simulink subsystem "VDBS14DOF"  (R2022a)
settings: Solver=VariableStepAuto  StartTime=0.0  StopTime=10.0  RelTol=1e-3
undefined symbols (not defined in the file or in its folder): egoActorID, max_ac, max_dc
settings Model: Creator=The MathWorks, Inc.  LastModifiedBy=The MathWorks, Inc.
settings SolverCC: MaxZcPerStep=1
settings DebuggingCC: UnconnectedInputMsg=warning  UnconnectedOutputMsg=warning  UnconnectedLineMsg=warning
settings RTWCC: DLArmComputeVersion=19.05

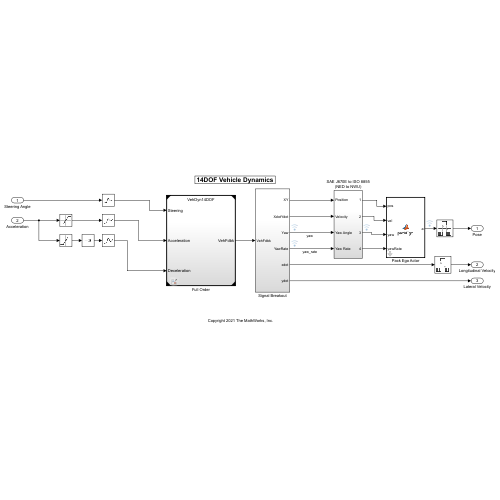
[thumbnail: Simulink's stored preview of the top-level diagram]
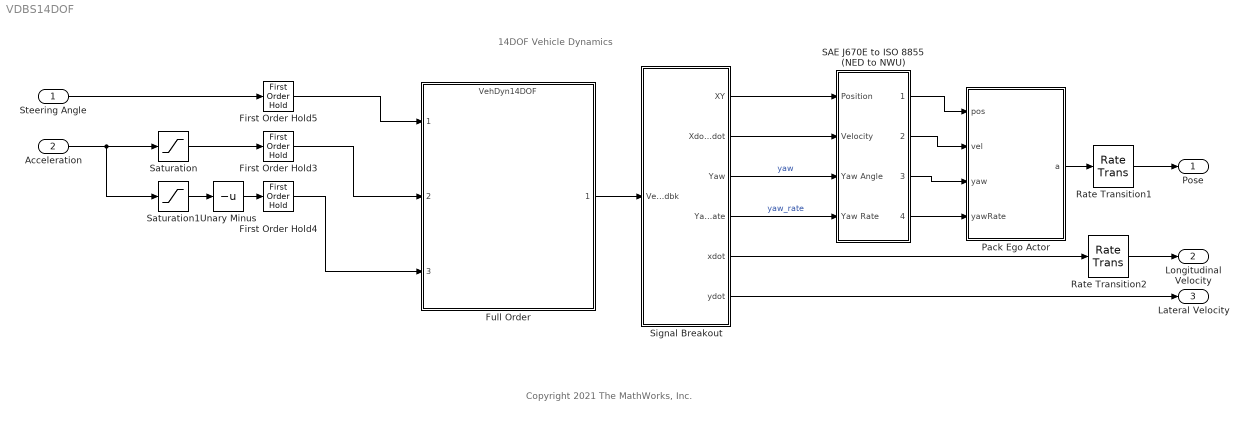
== system VDBS14DOF ==
  note: 14DOF Vehicle Dynamics
  note: Copyright 2021 The MathWorks, Inc.
  Steering Angle : Inport  Unit=rad
  Acceleration : Inport  Port=2  Unit=m/s^2
  First Order Hold3 : FirstOrderHold  ErrorTolerance=inf
  First Order Hold4 : FirstOrderHold  ErrorTolerance=inf
  First Order Hold5 : FirstOrderHold  ErrorTolerance=.1  AllowContinuousInput=on
  Full Order : ModelReference  ModelNameDialog=VehDyn14DOF  ModelReferenceVersion=3.5
  Pack Ego Actor : MATLAB Function  TreatAsAtomicUnit=on  mask{egoActorID=egoActorID}
      mask prompts: egoActorID "Ego Actor ID"
  Rate Transition1 : RateTransition  OutPortSampleTime=Ts
  Rate Transition2 : RateTransition  OutPortSampleTime=Ts
  SAE J670E to ISO 8855 (NED to NWU) : Subsystem
  Saturation : Saturate  UpperLimit=max_ac  LowerLimit=0
  Saturation1 : Saturate  UpperLimit=0  LowerLimit=max_dc
  Signal Breakout : Subsystem
  Unary Minus : UnaryMinus
  Pose : Outport  VectorParamsAs1DForOutWhenUnconnected=off
  Longitudinal Velocity : Outport  Port=2  Unit=m/s  VectorParamsAs1DForOutWhenUnconnected=off
  Lateral Velocity : Outport  Port=3  Unit=m/s  VectorParamsAs1DForOutWhenUnconnected=off
  wires:
  Acceleration/1 -> Saturation/1, Saturation1/1
  Saturation1/1 -> Unary Minus/1
  Signal Breakout/6(ydot) -> Lateral Velocity/1
  Rate Transition1/1 -> Pose/1
  Full Order/1 -> Signal Breakout/1(VehFdbk)
  Signal Breakout/1(XY) -> SAE J670E to ISO 8855 (NED to NWU)/1(Position)
  Signal Breakout/2(XdotYdot) -> SAE J670E to ISO 8855 (NED to NWU)/2(Velocity)
  Signal Breakout/3(Yaw) -> SAE J670E to ISO 8855 (NED to NWU)/3(Yaw Angle)  "yaw"
  Signal Breakout/4(YawRate) -> SAE J670E to ISO 8855 (NED to NWU)/4(Yaw Rate)  "yaw_rate"
  Pack Ego Actor/1(a) -> Rate Transition1/1
  SAE J670E to ISO 8855 (NED to NWU)/1(1) -> Pack Ego Actor/1(pos)
  SAE J670E to ISO 8855 (NED to NWU)/2(2) -> Pack Ego Actor/2(vel)
  SAE J670E to ISO 8855 (NED to NWU)/3(3) -> Pack Ego Actor/3(yaw)
  SAE J670E to ISO 8855 (NED to NWU)/4(4) -> Pack Ego Actor/4(yawRate)
  Signal Breakout/5(xdot) -> Rate Transition2/1
  Rate Transition2/1 -> Longitudinal Velocity/1
  Steering Angle/1 -> First Order Hold5/1
  Unary Minus/1 -> First Order Hold4/1
  Saturation/1 -> First Order Hold3/1
  First Order Hold5/1 -> Full Order/1
  First Order Hold4/1 -> Full Order/3
  First Order Hold3/1 -> Full Order/2

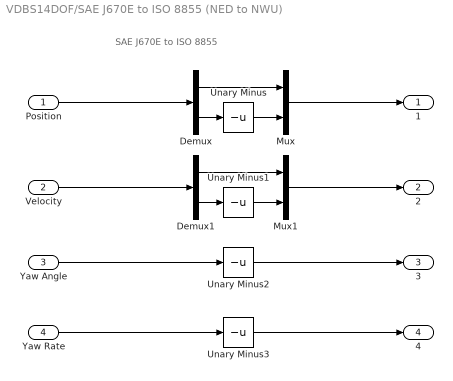
== system VDBS14DOF/SAE J670E to ISO 8855 (NED to NWU) ==
  note: SAE J670E to ISO 8855
  Position : Inport  Unit=m
  Velocity : Inport  Port=2  Unit=m/s
  Yaw Angle : Inport  Port=3  Unit=deg
  Yaw Rate : Inport  Port=4  Unit=deg/s
  Demux : Demux  Outputs=2
  Demux1 : Demux  Outputs=2
  Mux : Mux  Inputs=2
  Mux1 : Mux  Inputs=2
  Unary Minus{,1..3} (4 alike) : UnaryMinus
  1 : Outport  VectorParamsAs1DForOutWhenUnconnected=off
  2 : Outport  Port=2  VectorParamsAs1DForOutWhenUnconnected=off
  3 : Outport  Port=3  VectorParamsAs1DForOutWhenUnconnected=off
  4 : Outport  Port=4  VectorParamsAs1DForOutWhenUnconnected=off
  wires:
  Unary Minus3/1 -> 4/1
  Unary Minus2/1 -> 3/1
  Velocity/1 -> Demux1/1
  Position/1 -> Demux/1
  Mux/1 -> 1/1
  Mux1/1 -> 2/1
  Demux1/1 -> Mux1/1
  Demux1/2 -> Unary Minus1/1
  Unary Minus1/1 -> Mux1/2
  Unary Minus/1 -> Mux/2
  Demux/2 -> Unary Minus/1
  Demux/1 -> Mux/1
  Yaw Angle/1 -> Unary Minus2/1
  Yaw Rate/1 -> Unary Minus3/1

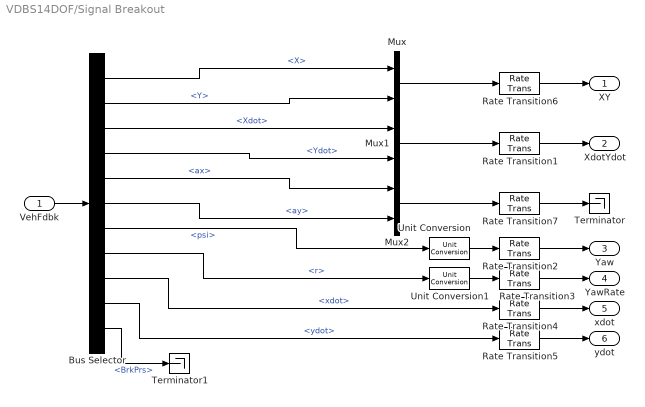
== system VDBS14DOF/Signal Breakout ==
  VehFdbk : Inport
  Bus Selector : BusSelector  OutputSignals=Body.InertFrm.Geom.Disp.X,Body.InertFrm.Geom.Disp.Y,Body.InertFrm.Geom.Vel.Xdot,Body.InertFrm.Geom.Vel.Ydot,Body.BdyFrm.Cg.Acc.ax,Body.BdyFrm.Cg.Acc.ay,Body.InertFrm.Cg.Ang.psi,Body.BdyFrm.Cg.AngVel.r,Body.BdyFrm.Cg.Vel.xdot,Body.BdyFrm.Cg.Vel.ydot,Driveline.BrkPrs
  Mux : Mux  Inputs=2
  Mux1 : Mux  Inputs=2
  Mux2 : Mux  Inputs=2
  Rate Transition{1..7} (7 alike) : RateTransition  OutPortSampleTime=Ts
  Terminator : Terminator
  Terminator1 : Terminator
  Unit Conversion : UnitConversion
  Unit Conversion1 : UnitConversion
  XY : Outport
  XdotYdot : Outport  Port=2
  Yaw : Outport  Port=3  Unit=deg
  YawRate : Outport  Port=4
  xdot : Outport  Port=5
  ydot : Outport  Port=6
  wires:
  Unit Conversion1/1 -> Rate Transition3/1
  Unit Conversion/1 -> Rate Transition2/1
  Mux/1 -> Rate Transition6/1
  Rate Transition2/1 -> Yaw/1
  Rate Transition4/1 -> xdot/1
  Mux1/1 -> Rate Transition1/1
  Rate Transition6/1 -> XY/1
  Mux2/1 -> Rate Transition7/1
  Rate Transition3/1 -> YawRate/1
  Bus Selector/9 -> Rate Transition4/1  "<xdot>"
  Rate Transition1/1 -> XdotYdot/1
  Rate Transition7/1 -> Terminator/1
  VehFdbk/1 -> Bus Selector/1
  Bus Selector/1 -> Mux/1  "<X>"
  Bus Selector/2 -> Mux/2  "<Y>"
  Bus Selector/3 -> Mux1/1  "<Xdot>"
  Bus Selector/4 -> Mux1/2  "<Ydot>"
  Bus Selector/5 -> Mux2/1  "<ax>"
  Bus Selector/6 -> Mux2/2  "<ay>"
  Bus Selector/8 -> Unit Conversion1/1  "<r>"
  Bus Selector/7 -> Unit Conversion/1  "<psi>"
  Bus Selector/10 -> Rate Transition5/1  "<ydot>"
  Rate Transition5/1 -> ydot/1
  Bus Selector/11 -> Terminator1/1  "<BrkPrs>"

== matlab function VDBS14DOF/Pack Ego Actor ==
  data: pos input; a output Bus: BusVehiclePose size=1; vel input; yaw input; yawRate input; egoActorID parameter
function a = packEgo(pos,vel,yaw,yawRate, egoActorID)
% Pack ego information into a single ego actor bus
%
% Important note:
% Output is a bus of type BusVehiclePose. This bus must match the bus 
% elements expected by Scenario Reader. You can view the 
% bus association using 'Edit Data' in the menu above.

a = struct(...
    'ActorID', egoActorID,...
    'Position', [pos(1) pos(2) 0], ...
    'Velocity', [vel(1) vel(2) 0], ...
    'Roll', 0, ...
    'Pitch', 0, ...
    'Yaw', yaw, ...
    'AngularVelocity', [0 0 yawRate]);
